simulink model "SYS2_1_with_reg"  (R2021b)
settings: Solver=ode3  StartTime=0.0  StopTime=0.1  FixedStep=1e-4  RelTol=1e-3
undefined symbols (not defined in the file or in its folder): Jn, K_bessel, K_butter, K_newton, ke, km, ku, L, R
settings Model: Creator=User  LastModifiedBy=vkad
settings SolverCC: AlgebraicLoopSolver=TrustRegion
settings DebuggingCC: SFMachineParentedDataDiag=warning

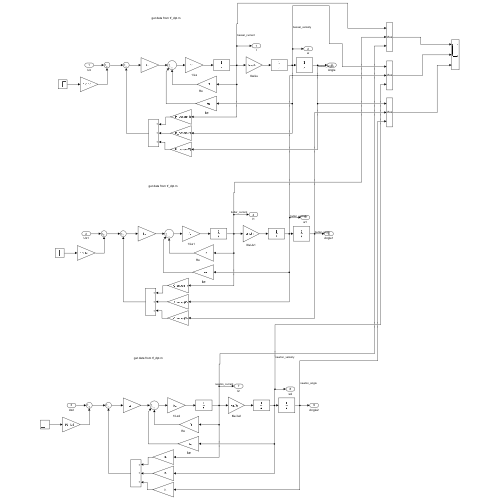
[thumbnail: Simulink's stored preview of the top-level diagram]
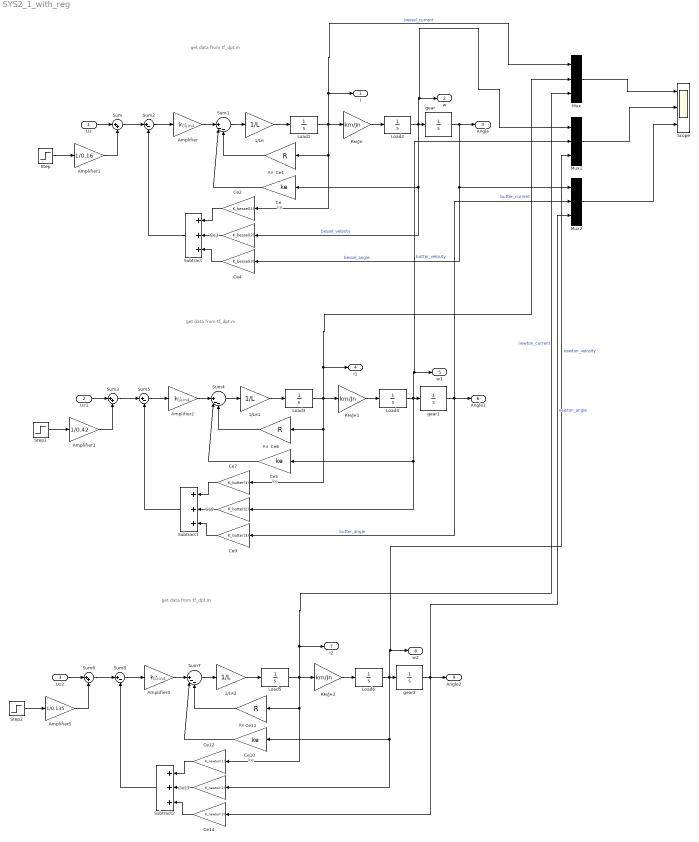
== system SYS2_1_with_reg ==
  note: get data from tf_dpt.m
  note: kе
  note: Rя
  note: Gain4
  note: get data from tf_dpt.m
  note: kе
  note: Rя
  note: Gain4
  note: get data from tf_dpt.m
  note: kе
  note: Rя
  note: Gain4
  Uz : Inport
  Uz1 : Inport  Port=2
  Uz2 : Inport  Port=3
  1/Lя : Gain  Gain=1/L
  1/Lя1 : Gain  Gain=1/L
  1/Lя2 : Gain  Gain=1/L
  Amplifier : Gain  Gain=ku
  Amplifier1 : Gain  Gain=1/0.16
  Amplifier2 : Gain  Gain=ku
  Amplifier3 : Gain  Gain=1/0.42
  Amplifier4 : Gain  Gain=ku
  Amplifier5 : Gain  Gain=1/0.135
  Ce : Gain  Gain=ke
  Ce1 : Gain  Gain=R
  Ce10 : Gain  Gain=ke
  Ce11 : Gain  Gain=R
  Ce12 : Gain  Gain=K_newton(1)
  Ce13 : Gain  Gain=K_newton(2)
  Ce14 : Gain  Gain=K_newton(3)
  Ce2 : Gain  Gain=K_bessel(1)
  Ce3 : Gain  Gain=K_bessel(2)
  Ce4 : Gain  Gain=K_bessel(3)
  Ce5 : Gain  Gain=ke
  Ce6 : Gain  Gain=R
  Ce7 : Gain  Gain=K_butter(1)
  Ce8 : Gain  Gain=K_butter(2)
  Ce9 : Gain  Gain=K_butter(3)
  Load{1..6} (6 alike) : TransferFcn  Denominator=[1 0]
  Mux : Mux  Inputs=3
  Mux1 : Mux  Inputs=3
  Mux2 : Mux  Inputs=3
  Scope : Scope  NumInputPorts=3
  Step : Step  Time=0  SampleTime=0
  Step1 : Step  Time=0  SampleTime=0
  Step2 : Step  Time=0  SampleTime=0
  Subtract : Sum  Inputs=+++
  Subtract1 : Sum  Inputs=+++
  Subtract2 : Sum  Inputs=+++
  Sum : Sum  Inputs=|++
  Sum1 : Sum  Inputs=||+--
  Sum2 : Sum  Inputs=|+-
  Sum3 : Sum  Inputs=|++
  Sum4 : Sum  Inputs=||+--
  Sum5 : Sum  Inputs=|+-
  Sum6 : Sum  Inputs=|++
  Sum7 : Sum  Inputs=||+--
  Sum8 : Sum  Inputs=|+-
  gear : TransferFcn  Numerator=1  Denominator=[1 0]
  gear1 : TransferFcn  Numerator=1  Denominator=[1 0]
  gear2 : TransferFcn  Numerator=1  Denominator=[1 0]
  Км/Jн : Gain  Gain=km/Jn
  Км/Jн1 : Gain  Gain=km/Jn
  Км/Jн2 : Gain  Gain=km/Jn
  I : Outport
  w : Outport  Port=2
  Angle : Outport  Port=3
  I1 : Outport  Port=4
  w1 : Outport  Port=5
  Angle1 : Outport  Port=6
  I2 : Outport  Port=7
  w2 : Outport  Port=8
  Angle2 : Outport  Port=9
  wires:
  Amplifier/1 -> Sum1/1
  Ce/1 -> Sum1/2
  Load2/1 -> Mux1/1, w/1, Ce3/1, Ce/1, gear/1  "bessel_velosity"
  Sum1/1 -> 1/Lя/1
  Uz/1 -> Sum/1
  1/Lя/1 -> Load1/1
  Ce1/1 -> Sum1/3
  Load1/1 -> Ce2/1, Ce1/1, Км/Jн/1, Mux/1, I/1  "bessel_current"
  Км/Jн/1 -> Load2/1
  Ce4/1 -> Subtract/3
  Subtract/1 -> Sum2/2
  Ce3/1 -> Subtract/2
  Ce2/1 -> Subtract/1
  gear/1 -> Mux2/1, Ce4/1, Angle/1  "bessel_angle"
  Sum/1 -> Sum2/1
  Sum2/1 -> Amplifier/1
  Step/1 -> Amplifier1/1
  Amplifier1/1 -> Sum/2
  Amplifier3/1 -> Sum3/2
  Step1/1 -> Amplifier3/1
  Sum5/1 -> Amplifier2/1
  Sum3/1 -> Sum5/1
  gear1/1 -> Mux2/2, Ce9/1, Angle1/1  "butter_angle"
  Ce7/1 -> Subtract1/1
  Ce8/1 -> Subtract1/2
  Subtract1/1 -> Sum5/2
  Ce9/1 -> Subtract1/3
  Км/Jн1/1 -> Load4/1
  Load3/1 -> Mux/2, I1/1, Км/Jн1/1, Ce6/1, Ce7/1  "butter_current"
  Ce6/1 -> Sum4/3
  1/Lя1/1 -> Load3/1
  Uz1/1 -> Sum3/1
  Sum4/1 -> 1/Lя1/1
  Load4/1 -> gear1/1, Ce5/1, Ce8/1, Mux1/2, w1/1  "butter_velosity"
  Ce5/1 -> Sum4/2
  Amplifier2/1 -> Sum4/1
  Amplifier4/1 -> Sum7/1
  Ce10/1 -> Sum7/2
  Load6/1 -> Mux1/3, w2/1, Ce13/1, Ce10/1, gear2/1  "newton_velosity"
  Sum7/1 -> 1/Lя2/1
  Uz2/1 -> Sum6/1
  1/Lя2/1 -> Load5/1
  Ce11/1 -> Sum7/3
  Load5/1 -> Ce12/1, Ce11/1, Км/Jн2/1, Mux/3, I2/1  "newton_current"
  Км/Jн2/1 -> Load6/1
  Ce14/1 -> Subtract2/3
  Subtract2/1 -> Sum8/2
  Ce13/1 -> Subtract2/2
  Ce12/1 -> Subtract2/1
  gear2/1 -> Mux2/3, Angle2/1, Ce14/1  "newton_angle"
  Sum6/1 -> Sum8/1
  Sum8/1 -> Amplifier4/1
  Step2/1 -> Amplifier5/1
  Amplifier5/1 -> Sum6/2
  Mux/1 -> Scope/1
  Mux1/1 -> Scope/2
  Mux2/1 -> Scope/3
